simulink model "Grafica_Simulink"  (R2020a)
settings: Solver=VariableStepAuto  StartTime=0.0  StopTime=180  RelTol=1e-3
settings Model: Creator=HP  LastModifiedBy=HP

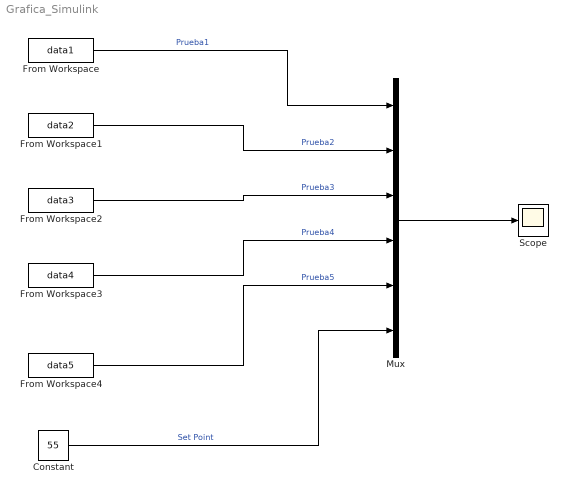
== system Grafica_Simulink ==
  Constant : Constant  Value=55
  From Workspace : FromWorkspace  VariableName=data1
  From Workspace1 : FromWorkspace  VariableName=data2
  From Workspace2 : FromWorkspace  VariableName=data3
  From Workspace3 : FromWorkspace  VariableName=data4
  From Workspace4 : FromWorkspace  VariableName=data5
  Mux : Mux  Inputs=6
  Scope : Scope
  wires:
  Mux/1 -> Scope/1
  From Workspace/1 -> Mux/1  "Prueba1"
  From Workspace1/1 -> Mux/2  "Prueba2"
  From Workspace2/1 -> Mux/3  "Prueba3"
  From Workspace3/1 -> Mux/4  "Prueba4"
  From Workspace4/1 -> Mux/5  "Prueba5"
  Constant/1 -> Mux/6  "Set Point"
